simulink model "simulation_w_switch_sln3"  (Simulink 10.1)
settings: Solver=VariableStepAuto  StartTime=0.0  StopTime=tTot  MaxStep=1e-5  RelTol=1e-5
PreLoadFcn:
  | syst_init
values from neighbouring files (symbols this model uses):
  Aij = Aconn-Aii    [syst_init.m]
  AL = blkdiag(DGU.ALi)    [syst_init.m]
  atk24 = [zeros(3,1); 0.1*rand(3,1)-0.05]    [syst_init.m]
  atk34 = [zeros(3,1); 0.1*rand(3,1)-0.05]    [syst_init.m]
  B = blkdiag(DGU.B)    [syst_init.m]
  bC = blkdiag(DGU.bC)    [syst_init.m]
  bF = blkdiag(DGU.bF)    [syst_init.m]
  bH = blkdiag(DGU.bH)    [syst_init.m]
  bigCyComm = [zeros(3,3)  eye(3) zeros(3,30) ... (first row only)    [syst_init.m]
  bKhat = blkdiag(DGU.bKhat)    [syst_init.m]
  DGU = stateDyn(DGU,6)    [syst_init.m]
  F = blkdiag(DGU.Fj)    [syst_init.m]
  H = blkdiag(DGU.Hj)    [syst_init.m]
  K = blkdiag(DGU.K)    [syst_init.m]
  Khat = blkdiag(DGU.Khat)    [syst_init.m]
  L = blkdiag(DGU.Li)    [syst_init.m]
  n = 3    [syst_init.m]
  N = 6    [syst_init.m]
  nMaxMeas = .01    (= 0.01)    [syst_init.m]
  rhoMax = nMaxMeas*repmat([ones(n-1,1);0],N,1)    [syst_init.m]
  T = blkdiag(DGU.Tj)    [syst_init.m]
  Ta = 8    [syst_init.m]
  Tc = 2    [syst_init.m]
  tSampData = 1e-3    (= 0.001)    [syst_init.m]
  Vs = 60    [syst_init.m]
  wMax = nMax*repmat([ones(n-1,1);0],N,1)+nMaxMeas*repmat([zeros(n-1,1);1],N,1)    [syst_init.m]
undefined symbols (not defined in the file or in its folder): epsilon0bar, integral_Loc, rLoc_bar
libraries: powerlib x136, powerlib_meascontrol x13
(part 3 of 4)

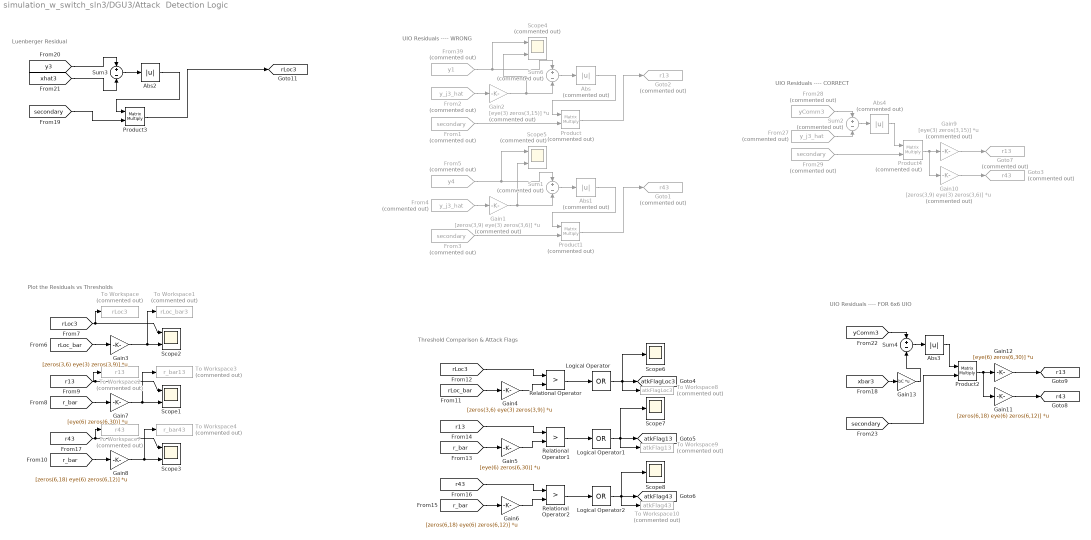
== system simulation_w_switch_sln3/DGU3/Attack  Detection Logic ==
  note: Luenberger Residual
  note: UIO Residuals ---- WRONG
  note: Threshold Comparison & Attack Flags
  note: Plot the Residuals vs Thresholds
  note: UIO Residuals ---- CORRECT
  note: UIO Residuals ---- FOR 6x6 UIO
  Abs : Abs  Commented=on
  Abs1 : Abs  Commented=on
  Abs2 : Abs
  Abs3 : Abs  ZeroCross=off
  Abs4 : Abs  Commented=on
  From1 : From  Commented=on  GotoTag=secondary  TagVisibility=global
  From2 : From  Commented=on  GotoTag=y_j3_hat  TagVisibility=global
  From27 : From  Commented=on  GotoTag=y_j3_hat  TagVisibility=global
  From28 : From  Commented=on  GotoTag=yComm3  TagVisibility=global
  From29 : From  Commented=on  GotoTag=secondary  TagVisibility=global
  From3 : From  Commented=on  GotoTag=secondary  TagVisibility=global
  From39 : From  Commented=on  GotoTag=y1  TagVisibility=global
  From4 : From  Commented=on  GotoTag=y_j3_hat  TagVisibility=global
  From5 : From  Commented=on  GotoTag=y4  TagVisibility=global
  Gain1 : Gain  Commented=on  Gain=[zeros(3,9) eye(3) zeros(3,6)]  Multiplication=Matrix(K*u) (u vector)
  Gain10 : Gain  Commented=on  Gain=[zeros(3,9) eye(3) zeros(3,6)]  Multiplication=Matrix(K*u) (u vector)
  Gain11 : Gain  Gain=[zeros(6,18) eye(6) zeros(6,12)]  Multiplication=Matrix(K*u) (u vector)
  Gain12 : Gain  Gain=[eye(6) zeros(6,30)]  Multiplication=Matrix(K*u) (u vector)
  Gain13 : Gain  Gain=bC  Multiplication=Matrix(K*u) (u vector)
  Gain2 : Gain  Commented=on  Gain=[eye(3) zeros(3,15)]  Multiplication=Matrix(K*u) (u vector)
  Gain3 : Gain  Gain=[zeros(3,6) eye(3) zeros(3,9)]  Multiplication=Matrix(K*u) (u vector)
  Gain4 : Gain  Gain=[zeros(3,6) eye(3) zeros(3,9)]  Multiplication=Matrix(K*u) (u vector)
  Gain5 : Gain  Gain=[eye(6) zeros(6,30)]  Multiplication=Matrix(K*u) (u vector)
  Gain6 : Gain  Gain=[zeros(6,18) eye(6) zeros(6,12)]  Multiplication=Matrix(K*u) (u vector)
  Gain7 : Gain  Gain=[eye(6) zeros(6,30)]  Multiplication=Matrix(K*u) (u vector)
  Gain8 : Gain  Gain=[zeros(6,18) eye(6) zeros(6,12)]  Multiplication=Matrix(K*u) (u vector)
  Gain9 : Gain  Commented=on  Gain=[eye(3) zeros(3,15)]  Multiplication=Matrix(K*u) (u vector)
  Goto1 : Goto  Commented=on  GotoTag=r43  TagVisibility=global
  Goto2 : Goto  Commented=on  GotoTag=r13  TagVisibility=global
  Goto3 : Goto  Commented=on  GotoTag=r43  TagVisibility=global
  Goto7 : Goto  Commented=on  GotoTag=r13  TagVisibility=global
  Logical Operator : Logic  Operator=OR  Inputs=1  AllPortsSameDT=off  OutDataTypeStr=boolean
  Logical Operator1 : Logic  Operator=OR  Inputs=1  AllPortsSameDT=off  OutDataTypeStr=boolean
  Logical Operator2 : Logic  Operator=OR  Inputs=1  AllPortsSameDT=off  OutDataTypeStr=boolean
  Product : Product  Commented=on  Multiplication=Matrix(*)
  Product1 : Product  Commented=on  Multiplication=Matrix(*)
  Product2 : Product  Multiplication=Matrix(*)
  Product3 : Product  Multiplication=Matrix(*)
  Product4 : Product  Commented=on  Multiplication=Matrix(*)
  Relational Operator : RelationalOperator  Operator=>  OutDataTypeStr=boolean  RndMeth=Simplest
  Relational Operator1 : RelationalOperator  Operator=>  OutDataTypeStr=boolean  RndMeth=Simplest
  Relational Operator2 : RelationalOperator  Operator=>  OutDataTypeStr=boolean  RndMeth=Simplest
  Scope1 : Scope  NumInputPorts=2
  Scope2 : Scope  NumInputPorts=2
  Scope3 : Scope  NumInputPorts=2
  Scope4 : Scope  Commented=on  NumInputPorts=2
  Scope5 : Scope  Commented=on  NumInputPorts=2
  Scope6 : Scope
  Scope7 : Scope
  Scope8 : Scope
  Sum1 : Sum  Commented=on  Inputs=+|-
  Sum2 : Sum  Commented=on  Inputs=+|-
  Sum3 : Sum  Inputs=+|-
  Sum4 : Sum  Inputs=+|-
  Sum6 : Sum  Commented=on  Inputs=+|-
  To Workspace : ToWorkspace  Commented=on  VariableName=rLoc3  SaveFormat=Timeseries  SampleTime=tSampData
  To Workspace1 : ToWorkspace  Commented=on  VariableName=rLoc_bar3  SaveFormat=Timeseries  SampleTime=tSampData
  To Workspace10 : ToWorkspace  Commented=on  VariableName=atkFlag43  SaveFormat=Timeseries  SampleTime=tSampData
  To Workspace2 : ToWorkspace  Commented=on  VariableName=r13  SaveFormat=Timeseries  SampleTime=tSampData
  To Workspace3 : ToWorkspace  Commented=on  VariableName=r_bar13  SaveFormat=Timeseries  SampleTime=tSampData
  To Workspace4 : ToWorkspace  Commented=on  VariableName=r_bar43  SaveFormat=Timeseries  SampleTime=tSampData
  To Workspace7 : ToWorkspace  Commented=on  VariableName=r43  SaveFormat=Timeseries  SampleTime=tSampData
  To Workspace8 : ToWorkspace  Commented=on  VariableName=atkFlagLoc3  SaveFormat=Timeseries  SampleTime=tSampData
  To Workspace9 : ToWorkspace  Commented=on  VariableName=atkFlag13  SaveFormat=Timeseries  SampleTime=tSampData
  tag scope: atkFlag13=global, atkFlag43=global, atkFlagLoc3=global, r13=global, r43=global, rLoc3=global
  wires:
  Abs2/1 -> Product3/1
  [secondary] -> Product3/2
  [xhat3] -> Sum3/2
  Sum3/1 -> Abs2/1
  Product3/1 -> [rLoc3]
  [y3] -> Sum3/1
  Gain2/1 -> Scope4/2, Sum6/2
  Sum1/1 -> Abs1/1
  Sum6/1 -> Abs/1
  Product1/1 -> Goto1/1
  Abs1/1 -> Product1/1
  From5/1 -> Scope5/1, Sum1/1
  From2/1 -> Gain2/1
  From4/1 -> Gain1/1
  From1/1 -> Product/2
  Gain1/1 -> Scope5/2, Sum1/2
  From3/1 -> Product1/2
  Abs/1 -> Product/1
  Product/1 -> Goto2/1
  From39/1 -> Scope4/1, Sum6/1
  Relational Operator1/1 -> Logical Operator1/1
  [rLoc_bar] -> Gain4/1
  Logical Operator1/1 -> Scope7/1, To Workspace9/1, [atkFlag13]
  [rLoc3] -> Relational Operator/1
  Relational Operator/1 -> Logical Operator/1
  [r_bar] -> Gain5/1
  Gain5/1 -> Relational Operator1/2
  Logical Operator/1 -> Scope6/1, To Workspace8/1, [atkFlagLoc3]
  [r13] -> Relational Operator1/1
  Relational Operator2/1 -> Logical Operator2/1
  Gain4/1 -> Relational Operator/2
  Gain6/1 -> Relational Operator2/2
  [r43] -> Relational Operator2/1
  [r_bar] -> Gain6/1
  Logical Operator2/1 -> Scope8/1, To Workspace10/1, [atkFlag43]
  [r_bar] -> Gain8/1
  [r43] -> To Workspace7/1, Scope3/1
  [r13] -> To Workspace2/1, Scope1/1
  [r_bar] -> Gain7/1
  Gain7/1 -> To Workspace3/1, Scope1/2
  [rLoc_bar] -> Gain3/1
  Gain3/1 -> To Workspace1/1, Scope2/2
  Gain8/1 -> To Workspace4/1, Scope3/2
  [rLoc3] -> To Workspace/1, Scope2/1
  From29/1 -> Product4/2
  From27/1 -> Sum2/2
  From28/1 -> Sum2/1
  Sum2/1 -> Abs4/1
  Product4/1 -> Gain10/1, Gain9/1
  Abs4/1 -> Product4/1
  Gain9/1 -> Goto7/1
  Gain10/1 -> Goto3/1
  Gain11/1 -> [r43]
  Gain12/1 -> [r13]
  Abs3/1 -> Product2/1
  Product2/1 -> Gain12/1, Gain11/1
  Sum4/1 -> Abs3/1
  [yComm3] -> Sum4/1
  [secondary] -> Product2/2
  [xbar3] -> Gain13/1
  Gain13/1 -> Sum4/2

== system simulation_w_switch_sln3/DGU3/Luenberger  Observer ==
  Gain1 : Gain  Gain=bigCyComm  Multiplication=Matrix(K*u) (u vector)
  Gain17 : Gain  Gain=[DGU(3).B , DGU(3).Li , DGU(3).M , Aij(2*n+1:3*n,:)]  Multiplication=Matrix(K*u) (u vector)
  Gain18 : Gain  Gain=DGU(3).A-DGU(3).Li*DGU(3).C  Multiplication=Matrix(K*u) (u vector)
  Integrator4 : Integrator  ExternalReset=rising  InitialConditionSource=external  InitialCondition=[0;0;0]
  Mux : Mux  Inputs=5
  Product4 : Product  Multiplication=Matrix(*)
  Sum10 : Sum  Inputs=++|
  tag scope: xhat3=global
  wires:
  Product4/1 -> [xhat3]
  [Il3] -> Mux/3
  [y3] -> Integrator4/3, Mux/2
  [Vref3] -> Mux/4
  Gain17/1 -> Sum10/2
  Gain18/1 -> Sum10/1
  [secondary] -> Integrator4/2, Product4/2
  Mux/1 -> Gain17/1
  Sum10/1 -> Integrator4/1
  Integrator4/1 -> Product4/1, Gain18/1
  [Vt3] -> Mux/1
  [yComm3] -> Gain1/1
  Gain1/1 -> Mux/5

== system simulation_w_switch_sln3/DGU3/Primary  Voltage  Controller ==
  Gain1 : Gain  Gain=DGU(3).K  Multiplication=Matrix(K*u) (u vector)
  tag scope: Vt3d=global
  wires:
  Gain1/1 -> [Vt3d]
  [y3] -> Gain1/1

== system simulation_w_switch_sln3/DGU3/Secondary  Consensus Layer ==
  note: deltaV3
  Gain14 : Gain  Gain=DGU(3).kI
  Gain2 : Gain  Gain=repmat([0 0 0 0 1 0],1,6)  Multiplication=Matrix(K*u) (u vector)
  Gain8 : Gain  Gain=length(DGU(3).Ni)
  Integrator2 : Integrator  ExternalReset=rising
  Sum10 : Sum  Inputs=|+-
  Sum11 : Sum  Inputs=|++
  Switch2 : Switch  Criteria=u2 > Threshold  Threshold=0.1
  tag scope: Vref3=global
  wires:
  Gain8/1 -> Sum10/2
  [It3] -> Gain8/1
  Integrator2/1 -> Sum11/1
  [secondary] -> Integrator2/2, Switch2/2
  Gain2/1 -> Sum10/1
  [yComm3] -> Gain2/1
  Sum10/1 -> Gain14/1
  Gain14/1 -> Integrator2/1
  Switch2/1 -> [Vref3]
  Sum11/1 -> Switch2/1
  [Vref] -> Switch2/3, Sum11/2

== system simulation_w_switch_sln3/DGU3/Switching ==
  Divide : Product  Inputs=*/
  Logical Operator : Logic  Operator=NOT  AllPortsSameDT=off  OutDataTypeStr=boolean
  PWM Generator (DC-DC) : powerlib_meascontrol/Pulse & Signal Generators/PWM Generator (DC-DC)  Fsw=10000  Ts=0
  tag scope: SW_Buck_3=global, SW_Buck_3n=global, SW_Duty_3=global
  wires:
  [Vs3] -> Divide/2
  Logical Operator/1 -> [SW_Buck_3n]
  PWM Generator (DC-DC)/1 -> Logical Operator/1, [SW_Buck_3]
  Divide/1 -> [SW_Duty_3], PWM Generator (DC-DC)/1
  [Vt3d] -> Divide/1

== system simulation_w_switch_sln3/DGU3/UIO ==
  note: Single UIO for all neighbors of DGU 1 with Switched Inputs
  note: Calculated Switching Inputs
  note: 6x6 UIO for the states of DGUs with average dynamics
  Constant1 : Constant  Commented=on  Value=Vs
  Constant2 : Constant  Commented=on  Value=0.8132
  Divide : Product  Commented=on  Inputs=*/  Multiplication=Matrix(*)
  From5 : From  Commented=on  GotoTag=yComm3  TagVisibility=global
  From7 : From  Commented=on  GotoTag=yComm3  TagVisibility=global
  From8 : From  Commented=on  GotoTag=SW_yComm3  TagVisibility=global
  From9 : From  Commented=on  GotoTag=secondary  TagVisibility=global
  Gain15 : Gain  Gain=bH  Multiplication=Matrix(K*u) (u vector)
  Gain16 : Gain  Gain=inv(bC)-bH  Multiplication=Matrix(K*u) (u vector)
  Gain17 : Gain  Gain=bKhat  Multiplication=Matrix(K*u) (u vector)
  Gain18 : Gain  Gain=bF  Multiplication=Matrix(K*u) (u vector)
  Gain4 : Gain  Commented=on  Gain=K  Multiplication=Matrix(K*u) (u vector)
  Gain5 : Gain  Commented=on  Gain=[Khat T*B]  Multiplication=Matrix(K*u) (u vector)
  Gain6 : Gain  Commented=on  Gain=F  Multiplication=Matrix(K*u) (u vector)
  Gain7 : Gain  Commented=on  Gain=59.7999
  Gain8 : Gain  Commented=on  Gain=H  Multiplication=Matrix(K*u) (u vector)
  Gain9 : Gain  Commented=on  Gain=T  Multiplication=Matrix(K*u) (u vector)
  Goto : Goto  Commented=on  GotoTag=SW_yComm3  TagVisibility=global
  Goto3 : Goto  Commented=on  GotoTag=y_j3_hat  TagVisibility=global
  Goto4 : Goto  Commented=on  GotoTag=Duty_yComm3  TagVisibility=global
  Integrator1 : Integrator  Commented=on  ExternalReset=rising  InitialConditionSource=external
  Integrator4 : Integrator  ExternalReset=rising  InitialConditionSource=external  InitialCondition=[0;0;0]
  Mux3 : Mux  Commented=on  Inputs=2
  PWM Generator (DC-DC) : powerlib_meascontrol/Pulse & Signal Generators/PWM Generator (DC-DC)  Commented=on  Fsw=10000  Ts=0
  Product1 : Product  Commented=on  Multiplication=Matrix(*)
  Product4 : Product  Multiplication=Matrix(*)
  Sum10 : Sum  Inputs=++|
  Sum11 : Sum  Inputs=++|
  Sum2 : Sum  Commented=on  Inputs=++|
  Sum3 : Sum  Commented=on  Inputs=++|
  Sum4 : Sum  Commented=on  Inputs=|-+
  tag scope: xbar3=global
  wires:
  PWM Generator (DC-DC)/1 -> Goto/1
  Divide/1 -> Goto4/1, PWM Generator (DC-DC)/1
  Constant1/1 -> Divide/2
  Gain4/1 -> Divide/1
  From7/1 -> Gain4/1
  Constant2/1 -> Sum4/1
  From5/1 -> Gain8/1, Gain9/1, Mux3/1
  Sum3/1 -> Product1/1
  Gain5/1 -> Sum2/2
  Gain7/1 -> Sum4/2
  From8/1 -> Gain7/1
  Mux3/1 -> Gain5/1
  Gain8/1 -> Sum3/1
  Gain9/1 -> Integrator1/3
  From9/1 -> Integrator1/2, Product1/2
  Sum2/1 -> Integrator1/1
  Sum4/1 -> Mux3/2
  Integrator1/1 -> Sum3/2, Gain6/1
  Gain6/1 -> Sum2/1
  Product1/1 -> Goto3/1
  Gain17/1 -> Sum10/2
  Gain18/1 -> Sum10/1
  [secondary] -> Integrator4/2, Product4/2
  Product4/1 -> [xbar3]
  Integrator4/1 -> Sum11/2, Gain18/1
  Gain15/1 -> Sum11/1
  Sum10/1 -> Integrator4/1
  [yComm3] -> Gain16/1, Gain15/1, Gain17/1
  Gain16/1 -> Integrator4/3
  Sum11/1 -> Product4/1

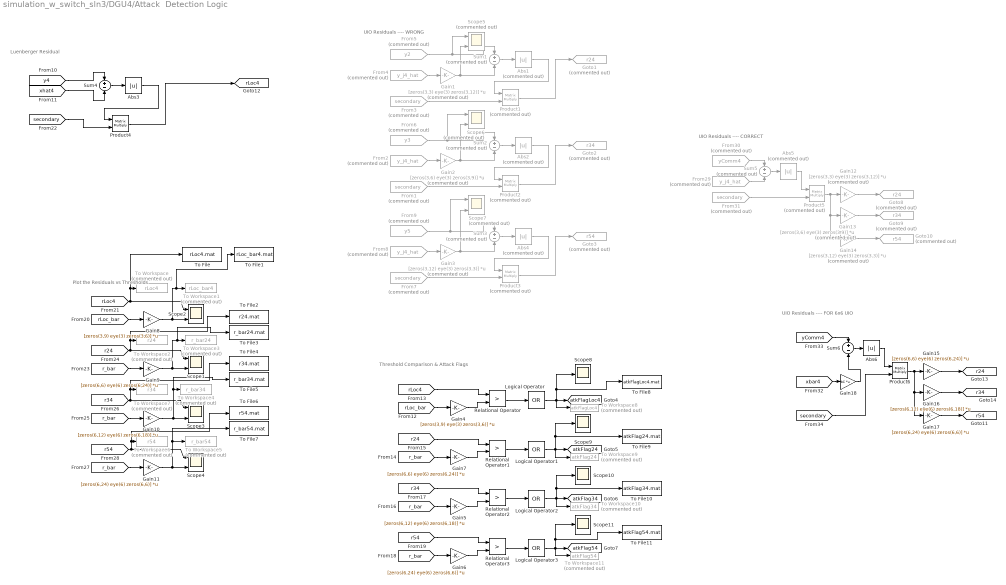
== system simulation_w_switch_sln3/DGU4/Attack  Detection Logic ==
  note: UIO Residuals ---- WRONG
  note: Luenberger Residual
  note: Threshold Comparison & Attack Flags
  note: Plot the Residuals vs Thresholds
  note: UIO Residuals ---- CORRECT
  note: UIO Residuals ---- FOR 6x6 UIO
  Abs{1..2,4..5} (4 alike) : Abs  Commented=on
  Abs3 : Abs
  Abs6 : Abs  ZeroCross=off
  From{1,3,7,31} (4 alike) : From  Commented=on  GotoTag=secondary  TagVisibility=global
  From{2,4,8,29} (4 alike) : From  Commented=on  GotoTag=y_j4_hat  TagVisibility=global
  From30 : From  Commented=on  GotoTag=yComm4  TagVisibility=global
  From5 : From  Commented=on  GotoTag=y2  TagVisibility=global
  From6 : From  Commented=on  GotoTag=y3  TagVisibility=global
  From9 : From  Commented=on  GotoTag=y5  TagVisibility=global
  Gain1 : Gain  Commented=on  Gain=[zeros(3,3) eye(3) zeros(3,12)]  Multiplication=Matrix(K*u) (u vector)
  Gain10 : Gain  Gain=[zeros(6,12) eye(6) zeros(6,18)]  Multiplication=Matrix(K*u) (u vector)
  Gain11 : Gain  Gain=[zeros(6,24) eye(6) zeros(6,6)]  Multiplication=Matrix(K*u) (u vector)
  Gain12 : Gain  Commented=on  Gain=[zeros(3,3) eye(3) zeros(3,12)]  Multiplication=Matrix(K*u) (u vector)
  Gain13 : Gain  Commented=on  Gain=[zeros(3,6) eye(3) zeros(3,9)]  Multiplication=Matrix(K*u) (u vector)
  Gain14 : Gain  Commented=on  Gain=[zeros(3,12) eye(3) zeros(3,3)]  Multiplication=Matrix(K*u) (u vector)
  Gain15 : Gain  Gain=[zeros(6,6) eye(6) zeros(6,24)]  Multiplication=Matrix(K*u) (u vector)
  Gain16 : Gain  Gain=[zeros(6,12) eye(6) zeros(6,18)]  Multiplication=Matrix(K*u) (u vector)
  Gain17 : Gain  Gain=[zeros(6,24) eye(6) zeros(6,6)]  Multiplication=Matrix(K*u) (u vector)
  Gain18 : Gain  Gain=bC  Multiplication=Matrix(K*u) (u vector)
  Gain2 : Gain  Commented=on  Gain=[zeros(3,6) eye(3) zeros(3,9)]  Multiplication=Matrix(K*u) (u vector)
  Gain3 : Gain  Commented=on  Gain=[zeros(3,12) eye(3) zeros(3,3)]  Multiplication=Matrix(K*u) (u vector)
  Gain4 : Gain  Gain=[zeros(3,9) eye(3) zeros(3,6)]  Multiplication=Matrix(K*u) (u vector)
  Gain5 : Gain  Gain=[zeros(6,12) eye(6) zeros(6,18)]  Multiplication=Matrix(K*u) (u vector)
  Gain6 : Gain  Gain=[zeros(6,24) eye(6) zeros(6,6)]  Multiplication=Matrix(K*u) (u vector)
  Gain7 : Gain  Gain=[zeros(6,6) eye(6) zeros(6,24)]  Multiplication=Matrix(K*u) (u vector)
  Gain8 : Gain  Gain=[zeros(3,9) eye(3) zeros(3,6)]  Multiplication=Matrix(K*u) (u vector)
  Gain9 : Gain  Gain=[zeros(6,6) eye(6) zeros(6,24)]  Multiplication=Matrix(K*u) (u vector)
  Goto1 : Goto  Commented=on  GotoTag=r24  TagVisibility=global
  Goto10 : Goto  Commented=on  GotoTag=r54  TagVisibility=global
  Goto2 : Goto  Commented=on  GotoTag=r34  TagVisibility=global
  Goto3 : Goto  Commented=on  GotoTag=r54  TagVisibility=global
  Goto8 : Goto  Commented=on  GotoTag=r24  TagVisibility=global
  Goto9 : Goto  Commented=on  GotoTag=r34  TagVisibility=global
  Logical Operator{,1..3} (4 alike) : Logic  Operator=OR  Inputs=1  AllPortsSameDT=off  OutDataTypeStr=boolean
  Product{1..3,5} (4 alike) : Product  Commented=on  Multiplication=Matrix(*)
  Product4 : Product  Multiplication=Matrix(*)
  Product6 : Product  Multiplication=Matrix(*)
  Relational Operator{,1..3} (4 alike) : RelationalOperator  Operator=>  OutDataTypeStr=boolean  RndMeth=Simplest
  Scope{1..4} (4 alike) : Scope  NumInputPorts=2
  Scope{8..11} (4 alike) : Scope
  Scope5 : Scope  Commented=on  NumInputPorts=2
  Scope6 : Scope  Commented=on  NumInputPorts=2
  Scope7 : Scope  Commented=on  NumInputPorts=2
  Sum{1..3,5} (4 alike) : Sum  Commented=on  Inputs=+|-
  Sum4 : Sum  Inputs=+|-
  Sum6 : Sum  Inputs=+|-
  To File : ToFile  Filename=rLoc4.mat  MatrixName=rLoc4  SaveFormat=Timeseries  SampleTime=tSampData
  To File1 : ToFile  Filename=rLoc_bar4.mat  MatrixName=rLoc_bar4  SaveFormat=Timeseries  SampleTime=tSampData
  To File10 : ToFile  Filename=atkFlag34.mat  MatrixName=atkFlag34  SaveFormat=Timeseries  SampleTime=tSampData
  To File11 : ToFile  Filename=atkFlag54.mat  MatrixName=atkFlag54  SaveFormat=Timeseries  SampleTime=tSampData
  To File2 : ToFile  Filename=r24.mat  MatrixName=r24  SaveFormat=Timeseries  SampleTime=tSampData
  To File3 : ToFile  Filename=r_bar24.mat  MatrixName=r_bar24  SaveFormat=Timeseries  SampleTime=tSampData
  To File4 : ToFile  Filename=r34.mat  MatrixName=r34  SaveFormat=Timeseries  SampleTime=tSampData
  To File5 : ToFile  Filename=r_bar34.mat  MatrixName=r_bar34  SaveFormat=Timeseries  SampleTime=tSampData
  To File6 : ToFile  Filename=r54.mat  MatrixName=r54  SaveFormat=Timeseries  SampleTime=tSampData
  To File7 : ToFile  Filename=r_bar54.mat  MatrixName=r_bar54  SaveFormat=Timeseries  SampleTime=tSampData
  To File8 : ToFile  Filename=atkFlagLoc4.mat  MatrixName=atkFlagLoc4  SaveFormat=Timeseries  SampleTime=tSampData
  To File9 : ToFile  Filename=atkFlag24.mat  MatrixName=atkFlag24  SaveFormat=Timeseries  SampleTime=tSampData
  To Workspace : ToWorkspace  Commented=on  VariableName=rLoc4  SaveFormat=Timeseries  SampleTime=tSampData
  To Workspace1 : ToWorkspace  Commented=on  VariableName=rLoc_bar4  SaveFormat=Timeseries  SampleTime=tSampData
  To Workspace10 : ToWorkspace  Commented=on  VariableName=atkFlag34  SaveFormat=Timeseries  SampleTime=tSampData
  To Workspace11 : ToWorkspace  Commented=on  VariableName=atkFlag54  SaveFormat=Timeseries  SampleTime=tSampData
  To Workspace2 : ToWorkspace  Commented=on  VariableName=r24  SaveFormat=Timeseries  SampleTime=tSampData
  To Workspace3 : ToWorkspace  Commented=on  VariableName=r_bar24  SaveFormat=Timeseries  SampleTime=tSampData
  To Workspace4 : ToWorkspace  Commented=on  VariableName=r_bar34  SaveFormat=Timeseries  SampleTime=tSampData
  To Workspace5 : ToWorkspace  Commented=on  VariableName=r_bar54  SaveFormat=Timeseries  SampleTime=tSampData
  To Workspace6 : ToWorkspace  Commented=on  VariableName=r54  SaveFormat=Timeseries  SampleTime=tSampData
  To Workspace7 : ToWorkspace  Commented=on  VariableName=r34  SaveFormat=Timeseries  SampleTime=tSampData
  To Workspace8 : ToWorkspace  Commented=on  VariableName=atkFlagLoc4  SaveFormat=Timeseries  SampleTime=tSampData
  To Workspace9 : ToWorkspace  Commented=on  VariableName=atkFlag24  SaveFormat=Timeseries  SampleTime=tSampData
  tag scope: atkFlag24=global, atkFlag34=global, atkFlag54=global, atkFlagLoc4=global, r24=global, r34=global, r54=global, rLoc4=global
  wires:
  [secondary] -> Product4/2
  Product4/1 -> [rLoc4]
  Abs3/1 -> Product4/1
  [y4] -> Sum4/1
  Sum4/1 -> Abs3/1
  [xhat4] -> Sum4/2
  Gain1/1 -> Scope5/2, Sum1/2
  Abs1/1 -> Product1/1
  Product1/1 -> Goto1/1
  From3/1 -> Product1/2
  Sum1/1 -> Abs1/1
  From4/1 -> Gain1/1
  From6/1 -> Scope6/1, Sum2/1
  Abs2/1 -> Product2/1
  From1/1 -> Product2/2
  Product2/1 -> Goto2/1
  Gain2/1 -> Scope6/2, Sum2/2
  From2/1 -> Gain2/1
  Sum2/1 -> Abs2/1
  From9/1 -> Scope7/1, Sum3/1
  Abs4/1 -> Product3/1
  From7/1 -> Product3/2
  Product3/1 -> Goto3/1
  Gain3/1 -> Scope7/2, Sum3/2
  From8/1 -> Gain3/1
  Sum3/1 -> Abs4/1
  Logical Operator3/1 -> To Workspace11/1, Scope11/1, To File11/1, [atkFlag54]
  Relational Operator1/1 -> Logical Operator1/1
  [rLoc_bar] -> Gain4/1
  [r_bar] -> Gain6/1
  Logical Operator1/1 -> To Workspace9/1, To File9/1, Scope9/1, [atkFlag24]
  [r54] -> Relational Operator3/1
  [rLoc4] -> Relational Operator/1
  Relational Operator/1 -> Logical Operator/1
  Gain6/1 -> Relational Operator3/2
  [r_bar] -> Gain7/1
  Gain7/1 -> Relational Operator1/2
  Logical Operator/1 -> To Workspace8/1, To File8/1, Scope8/1, [atkFlagLoc4]
  Relational Operator3/1 -> Logical Operator3/1
  [r24] -> Relational Operator1/1
  Relational Operator2/1 -> Logical Operator2/1
  Gain4/1 -> Relational Operator/2
  Gain5/1 -> Relational Operator2/2
  [r34] -> Relational Operator2/1
  [r_bar] -> Gain5/1
  Logical Operator2/1 -> To Workspace10/1, Scope10/1, To File10/1, [atkFlag34]
  [rLoc_bar] -> Gain8/1
  [r_bar] -> Gain9/1
  [r54] -> To File6/1, To Workspace6/1, Scope4/1
  [r_bar] -> Gain10/1
  Gain11/1 -> To File7/1, To Workspace5/1, Scope4/2
  [rLoc4] -> To File/1, To Workspace/1, Scope2/1
  [r_bar] -> Gain11/1
  Gain9/1 -> To File3/1, To Workspace3/1, Scope1/2
  [r34] -> To File4/1, To Workspace7/1, Scope3/1
  Gain10/1 -> To File5/1, To Workspace4/1, Scope3/2
  Gain8/1 -> To File1/1, To Workspace1/1, Scope2/2
  [r24] -> To File2/1, To Workspace2/1, Scope1/1
  From5/1 -> Scope5/1, Sum1/1
  From31/1 -> Product5/2
  From29/1 -> Sum5/2
  From30/1 -> Sum5/1
  Sum5/1 -> Abs5/1
  Product5/1 -> Gain12/1, Gain14/1, Gain13/1
  Abs5/1 -> Product5/1
  Gain14/1 -> Goto10/1
  Gain13/1 -> Goto9/1
  Gain12/1 -> Goto8/1
  Gain15/1 -> [r24]
  Gain16/1 -> [r34]
  Gain17/1 -> [r54]
  Abs6/1 -> Product6/1
  Product6/1 -> Gain16/1, Gain17/1, Gain15/1
  Sum6/1 -> Abs6/1
  [yComm4] -> Sum6/1
  [secondary] -> Product6/2
  [xbar4] -> Gain18/1
  Gain18/1 -> Sum6/2

== system simulation_w_switch_sln3/DGU4/Luenberger  Observer ==
  Gain1 : Gain  Gain=bigCyComm  Multiplication=Matrix(K*u) (u vector)
  Gain17 : Gain  Gain=[DGU(4).B , DGU(4).Li , DGU(4).M , Aij(3*n+1:4*n,:)]  Multiplication=Matrix(K*u) (u vector)
  Gain18 : Gain  Gain=DGU(4).A-DGU(4).Li*DGU(4).C  Multiplication=Matrix(K*u) (u vector)
  Integrator4 : Integrator  ExternalReset=rising  InitialConditionSource=external  InitialCondition=[0;0;0]
  Mux : Mux  Inputs=5
  Product4 : Product  Multiplication=Matrix(*)
  Sum10 : Sum  Inputs=++|
  tag scope: xhat4=global
  wires:
  Product4/1 -> [xhat4]
  [Il4] -> Mux/3
  [y4] -> Integrator4/3, Mux/2
  [Vref4] -> Mux/4
  Gain17/1 -> Sum10/2
  Gain18/1 -> Sum10/1
  [secondary] -> Integrator4/2, Product4/2
  Mux/1 -> Gain17/1
  Sum10/1 -> Integrator4/1
  Integrator4/1 -> Product4/1, Gain18/1
  [Vt4] -> Mux/1
  [yComm4] -> Gain1/1
  Gain1/1 -> Mux/5

== system simulation_w_switch_sln3/DGU4/Primary  Voltage  Controller ==
  Gain1 : Gain  Gain=DGU(4).K  Multiplication=Matrix(K*u) (u vector)
  tag scope: Vt4d=global
  wires:
  Gain1/1 -> [Vt4d]
  [y4] -> Gain1/1

== system simulation_w_switch_sln3/DGU4/Secondary Consensus Layer ==
  note: deltaV4
  Gain15 : Gain  Gain=DGU(4).kI
  Gain3 : Gain  Gain=repmat([0 0 0 0 1 0],1,6)  Multiplication=Matrix(K*u) (u vector)
  Gain9 : Gain  Gain=length(DGU(4).Ni)
  Integrator3 : Integrator  ExternalReset=rising
  Sum12 : Sum  Inputs=|+-
  Sum13 : Sum  Inputs=|++
  Switch3 : Switch  Criteria=u2 > Threshold  Threshold=0.1
  tag scope: Vref4=global
  wires:
  Gain3/1 -> Sum12/1
  Switch3/1 -> [Vref4]
  Integrator3/1 -> Sum13/1
  [It4] -> Gain9/1
  Sum12/1 -> Gain15/1
  Sum13/1 -> Switch3/1
  Gain15/1 -> Integrator3/1
  [secondary] -> Integrator3/2, Switch3/2
  [Vref] -> Switch3/3, Sum13/2
  [yComm4] -> Gain3/1
  Gain9/1 -> Sum12/2

== system simulation_w_switch_sln3/DGU4/Switching ==
  Divide : Product  Inputs=*/
  Logical Operator : Logic  Operator=NOT  AllPortsSameDT=off  OutDataTypeStr=boolean
  PWM Generator (DC-DC) : powerlib_meascontrol/Pulse & Signal Generators/PWM Generator (DC-DC)  Fsw=10000  Ts=0
  tag scope: SW_Buck_4=global, SW_Buck_4n=global, SW_Duty_4=global
  wires:
  [Vs4] -> Divide/2
  Logical Operator/1 -> [SW_Buck_4n]
  PWM Generator (DC-DC)/1 -> Logical Operator/1, [SW_Buck_4]
  Divide/1 -> [SW_Duty_4], PWM Generator (DC-DC)/1
  [Vt4d] -> Divide/1

== system simulation_w_switch_sln3/DGU4/UIO ==
  note: Single UIO for all neighbors of DGU 1 with Switched Inputs
  note: Calculated Switching Inputs
  note: 6x6 UIO for the states of DGUs with average dynamics
  Constant1 : Constant  Commented=on  Value=Vs
  Constant2 : Constant  Commented=on  Value=0.8132
  Divide : Product  Commented=on  Inputs=*/  Multiplication=Matrix(*)
  From1 : From  Commented=on  GotoTag=u_SW_a2  TagVisibility=global
  From5 : From  Commented=on  GotoTag=yComm4  TagVisibility=global
  From7 : From  Commented=on  GotoTag=yComm4  TagVisibility=global
  From8 : From  Commented=on  GotoTag=SW_yComm4  TagVisibility=global
  From9 : From  Commented=on  GotoTag=secondary  TagVisibility=global
  Gain1 : Gain  Commented=on  Gain=[0 1 0 0 0 0]  Multiplication=Matrix(K*u) (u vector)
  Gain15 : Gain  Gain=bH  Multiplication=Matrix(K*u) (u vector)
  Gain16 : Gain  Gain=inv(bC)-bH  Multiplication=Matrix(K*u) (u vector)
  Gain17 : Gain  Gain=bKhat  Multiplication=Matrix(K*u) (u vector)
  Gain18 : Gain  Gain=bF  Multiplication=Matrix(K*u) (u vector)
  Gain4 : Gain  Commented=on  Gain=K  Multiplication=Matrix(K*u) (u vector)
  Gain5 : Gain  Commented=on  Gain=[Khat T*B]  Multiplication=Matrix(K*u) (u vector)
  Gain6 : Gain  Commented=on  Gain=F  Multiplication=Matrix(K*u) (u vector)
  Gain7 : Gain  Commented=on  Gain=59.7999
  Gain8 : Gain  Commented=on  Gain=H  Multiplication=Matrix(K*u) (u vector)
  Gain9 : Gain  Commented=on  Gain=T  Multiplication=Matrix(K*u) (u vector)
  Goto : Goto  Commented=on  GotoTag=SW_yComm4  TagVisibility=global
  Goto3 : Goto  Commented=on  GotoTag=y_j4_hat  TagVisibility=global
  Goto4 : Goto  Commented=on  GotoTag=Duty_yComm4  TagVisibility=global
  Integrator1 : Integrator  Commented=on  ExternalReset=rising  InitialConditionSource=external
  Integrator4 : Integrator  ExternalReset=rising  InitialConditionSource=external  InitialCondition=[0;0;0]
  Mux3 : Mux  Commented=on  Inputs=2
  PWM Generator (DC-DC) : powerlib_meascontrol/Pulse & Signal Generators/PWM Generator (DC-DC)  Commented=on  Fsw=10000  Ts=0
  Product1 : Product  Commented=on  Multiplication=Matrix(*)
  Product4 : Product  Multiplication=Matrix(*)
  Scope : Scope  Commented=on
  Sum1 : Sum  Commented=on  Inputs=+-|
  Sum10 : Sum  Inputs=++|
  Sum11 : Sum  Inputs=++|
  Sum2 : Sum  Commented=on  Inputs=++|
  Sum3 : Sum  Commented=on  Inputs=++|
  Sum4 : Sum  Commented=on  Inputs=|-+
  tag scope: xbar4=global
  wires:
  PWM Generator (DC-DC)/1 -> Goto/1
  Divide/1 -> Goto4/1, PWM Generator (DC-DC)/1
  Constant1/1 -> Divide/2
  Gain4/1 -> Divide/1
  From7/1 -> Gain4/1
  Constant2/1 -> Sum4/1
  From5/1 -> Gain8/1, Gain9/1, Mux3/1
  Sum3/1 -> Product1/1
  Gain5/1 -> Sum2/2
  Gain7/1 -> Sum4/2
  From8/1 -> Gain7/1
  Mux3/1 -> Gain5/1
  Gain8/1 -> Sum3/1
  Gain9/1 -> Integrator1/3
  From9/1 -> Integrator1/2, Product1/2
  Sum2/1 -> Integrator1/1
  Sum4/1 -> Gain1/1, Mux3/2
  Integrator1/1 -> Sum3/2, Gain6/1
  Gain6/1 -> Sum2/1
  Product1/1 -> Goto3/1
  Gain1/1 -> Sum1/1
  From1/1 -> Sum1/2
  Sum1/1 -> Scope/1
  Sum11/1 -> Product4/1
  Gain17/1 -> Sum10/2
  Gain16/1 -> Integrator4/3
  Sum10/1 -> Integrator4/1
  [yComm4] -> Gain16/1, Gain15/1, Gain17/1
  Gain18/1 -> Sum10/1
  Gain15/1 -> Sum11/1
  Product4/1 -> [xbar4]
  Integrator4/1 -> Sum11/2, Gain18/1
  [secondary] -> Integrator4/2, Product4/2

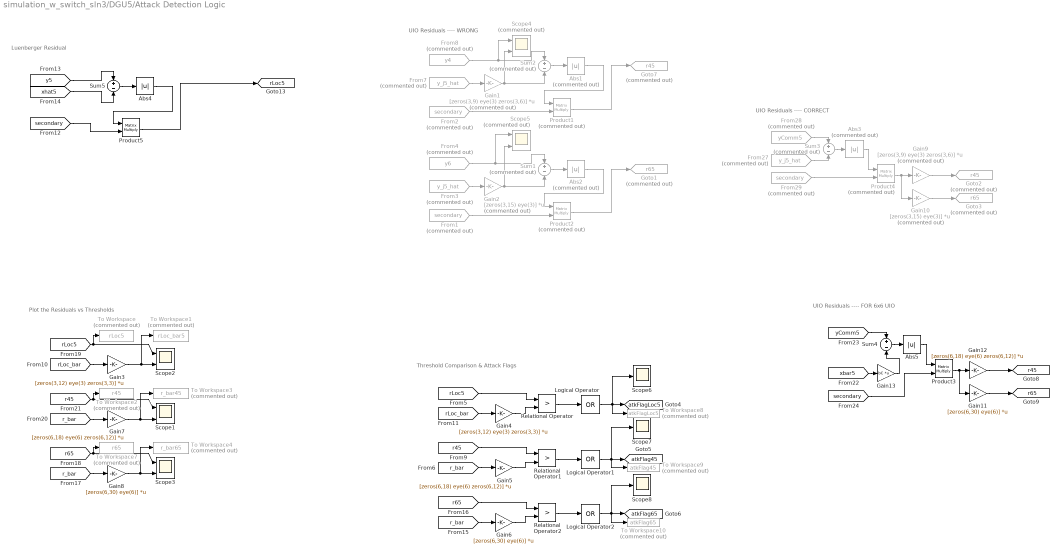
== system simulation_w_switch_sln3/DGU5/Attack Detection Logic ==
  note: UIO Residuals ---- WRONG
  note: Luenberger Residual
  note: Threshold Comparison & Attack Flags
  note: Plot the Residuals vs Thresholds
  note: UIO Residuals ---- CORRECT
  note: UIO Residuals ---- FOR 6x6 UIO
  Abs1 : Abs  Commented=on
  Abs2 : Abs  Commented=on
  Abs3 : Abs  Commented=on
  Abs4 : Abs
  Abs5 : Abs  ZeroCross=off
  From1 : From  Commented=on  GotoTag=secondary  TagVisibility=global
  From2 : From  Commented=on  GotoTag=secondary  TagVisibility=global
  From27 : From  Commented=on  GotoTag=y_j5_hat  TagVisibility=global
  From28 : From  Commented=on  GotoTag=yComm5  TagVisibility=global
  From29 : From  Commented=on  GotoTag=secondary  TagVisibility=global
  From3 : From  Commented=on  GotoTag=y_j5_hat  TagVisibility=global
  From4 : From  Commented=on  GotoTag=y6  TagVisibility=global
  From7 : From  Commented=on  GotoTag=y_j5_hat  TagVisibility=global
  From8 : From  Commented=on  GotoTag=y4  TagVisibility=global
  Gain1 : Gain  Commented=on  Gain=[zeros(3,9) eye(3) zeros(3,6)]  Multiplication=Matrix(K*u) (u vector)
  Gain10 : Gain  Commented=on  Gain=[zeros(3,15) eye(3)]  Multiplication=Matrix(K*u) (u vector)
  Gain11 : Gain  Gain=[zeros(6,30) eye(6)]  Multiplication=Matrix(K*u) (u vector)
  Gain12 : Gain  Gain=[zeros(6,18) eye(6) zeros(6,12)]  Multiplication=Matrix(K*u) (u vector)
  Gain13 : Gain  Gain=bC  Multiplication=Matrix(K*u) (u vector)
  Gain2 : Gain  Commented=on  Gain=[zeros(3,15) eye(3)]  Multiplication=Matrix(K*u) (u vector)
  Gain3 : Gain  Gain=[zeros(3,12) eye(3) zeros(3,3)]  Multiplication=Matrix(K*u) (u vector)
  Gain4 : Gain  Gain=[zeros(3,12) eye(3) zeros(3,3)]  Multiplication=Matrix(K*u) (u vector)
  Gain5 : Gain  Gain=[zeros(6,18) eye(6) zeros(6,12)]  Multiplication=Matrix(K*u) (u vector)
  Gain6 : Gain  Gain=[zeros(6,30) eye(6)]  Multiplication=Matrix(K*u) (u vector)
  Gain7 : Gain  Gain=[zeros(6,18) eye(6) zeros(6,12)]  Multiplication=Matrix(K*u) (u vector)
  Gain8 : Gain  Gain=[zeros(6,30) eye(6)]  Multiplication=Matrix(K*u) (u vector)
  Gain9 : Gain  Commented=on  Gain=[zeros(3,9) eye(3) zeros(3,6)]  Multiplication=Matrix(K*u) (u vector)
  Goto1 : Goto  Commented=on  GotoTag=r65  TagVisibility=global
  Goto2 : Goto  Commented=on  GotoTag=r45  TagVisibility=global
  Goto3 : Goto  Commented=on  GotoTag=r65  TagVisibility=global
  Goto7 : Goto  Commented=on  GotoTag=r45  TagVisibility=global
  Logical Operator : Logic  Operator=OR  Inputs=1  AllPortsSameDT=off  OutDataTypeStr=boolean
  Logical Operator1 : Logic  Operator=OR  Inputs=1  AllPortsSameDT=off  OutDataTypeStr=boolean
  Logical Operator2 : Logic  Operator=OR  Inputs=1  AllPortsSameDT=off  OutDataTypeStr=boolean
  Product1 : Product  Commented=on  Multiplication=Matrix(*)
  Product2 : Product  Commented=on  Multiplication=Matrix(*)
  Product3 : Product  Multiplication=Matrix(*)
  Product4 : Product  Commented=on  Multiplication=Matrix(*)
  Product5 : Product  Multiplication=Matrix(*)
  Relational Operator : RelationalOperator  Operator=>  OutDataTypeStr=boolean  RndMeth=Simplest
  Relational Operator1 : RelationalOperator  Operator=>  OutDataTypeStr=boolean  RndMeth=Simplest
  Relational Operator2 : RelationalOperator  Operator=>  OutDataTypeStr=boolean  RndMeth=Simplest
  Scope1 : Scope  NumInputPorts=2
  Scope2 : Scope  NumInputPorts=2
  Scope3 : Scope  NumInputPorts=2
  Scope4 : Scope  Commented=on  NumInputPorts=2
  Scope5 : Scope  Commented=on  NumInputPorts=2
  Scope6 : Scope
  Scope7 : Scope
  Scope8 : Scope
  Sum1 : Sum  Commented=on  Inputs=+|-
  Sum2 : Sum  Commented=on  Inputs=+|-
  Sum3 : Sum  Commented=on  Inputs=+|-
  Sum4 : Sum  Inputs=+|-
  Sum5 : Sum  Inputs=+|-
  To Workspace : ToWorkspace  Commented=on  VariableName=rLoc5  SaveFormat=Timeseries  SampleTime=tSampData
  To Workspace1 : ToWorkspace  Commented=on  VariableName=rLoc_bar5  SaveFormat=Timeseries  SampleTime=tSampData
  To Workspace10 : ToWorkspace  Commented=on  VariableName=atkFlag65  SaveFormat=Timeseries  SampleTime=tSampData
  To Workspace2 : ToWorkspace  Commented=on  VariableName=r45  SaveFormat=Timeseries  SampleTime=tSampData
  To Workspace3 : ToWorkspace  Commented=on  VariableName=r_bar45  SaveFormat=Timeseries  SampleTime=tSampData
  To Workspace4 : ToWorkspace  Commented=on  VariableName=r_bar65  SaveFormat=Timeseries  SampleTime=tSampData
  To Workspace7 : ToWorkspace  Commented=on  VariableName=r65  SaveFormat=Timeseries  SampleTime=tSampData
  To Workspace8 : ToWorkspace  Commented=on  VariableName=atkFlagLoc5  SaveFormat=Timeseries  SampleTime=tSampData
  To Workspace9 : ToWorkspace  Commented=on  VariableName=atkFlag45  SaveFormat=Timeseries  SampleTime=tSampData
  tag scope: atkFlag45=global, atkFlag65=global, atkFlagLoc5=global, r45=global, r65=global, rLoc5=global
  wires:
  [xhat5] -> Sum5/2
  Product5/1 -> [rLoc5]
  Sum5/1 -> Abs4/1
  [y5] -> Sum5/1
  Abs4/1 -> Product5/1
  [secondary] -> Product5/2
  Sum2/1 -> Abs1/1
  From2/1 -> Product1/2
  Gain1/1 -> Scope4/2, Sum2/2
  Product1/1 -> Goto7/1
  From7/1 -> Gain1/1
  Abs1/1 -> Product1/1
  From8/1 -> Scope4/1, Sum2/1
  Product2/1 -> Goto1/1
  From1/1 -> Product2/2
  From4/1 -> Scope5/1, Sum1/1
  From3/1 -> Gain2/1
  Sum1/1 -> Abs2/1
  Abs2/1 -> Product2/1
  Gain2/1 -> Sum1/2, Scope5/2
  Relational Operator1/1 -> Logical Operator1/1
  [rLoc_bar] -> Gain4/1
  Logical Operator1/1 -> To Workspace9/1, Scope7/1, [atkFlag45]
  [rLoc5] -> Relational Operator/1
  Relational Operator/1 -> Logical Operator/1
  [r_bar] -> Gain5/1
  Gain5/1 -> Relational Operator1/2
  Logical Operator/1 -> To Workspace8/1, Scope6/1, [atkFlagLoc5]
  [r45] -> Relational Operator1/1
  Relational Operator2/1 -> Logical Operator2/1
  Gain4/1 -> Relational Operator/2
  Gain6/1 -> Relational Operator2/2
  [r65] -> Relational Operator2/1
  [r_bar] -> Gain6/1
  Logical Operator2/1 -> To Workspace10/1, Scope8/1, [atkFlag65]
  Gain8/1 -> To Workspace4/1, Scope3/2
  [rLoc_bar] -> Gain3/1
  [r_bar] -> Gain8/1
  Gain3/1 -> To Workspace1/1, Scope2/2
  [r45] -> To Workspace2/1, Scope1/1
  [r_bar] -> Gain7/1
  Gain7/1 -> To Workspace3/1, Scope1/2
  [r65] -> To Workspace7/1, Scope3/1
  [rLoc5] -> To Workspace/1, Scope2/1
  From29/1 -> Product4/2
  From27/1 -> Sum3/2
  From28/1 -> Sum3/1
  Sum3/1 -> Abs3/1
  Product4/1 -> Gain9/1, Gain10/1
  Abs3/1 -> Product4/1
  Gain9/1 -> Goto2/1
  Gain10/1 -> Goto3/1
  Gain11/1 -> [r65]
  Gain12/1 -> [r45]
  Abs5/1 -> Product3/1
  Product3/1 -> Gain11/1, Gain12/1
  Sum4/1 -> Abs5/1
  [yComm5] -> Sum4/1
  [secondary] -> Product3/2
  Gain13/1 -> Sum4/2
  [xbar5] -> Gain13/1

== system simulation_w_switch_sln3/DGU5/Luenberger  Observer ==
  Gain1 : Gain  Gain=bigCyComm  Multiplication=Matrix(K*u) (u vector)
  Gain17 : Gain  Gain=[DGU(5).B , DGU(5).Li , DGU(5).M , Aij(4*n+1:5*n,:)]  Multiplication=Matrix(K*u) (u vector)
  Gain18 : Gain  Gain=DGU(5).A-DGU(5).Li*DGU(5).C  Multiplication=Matrix(K*u) (u vector)
  Integrator4 : Integrator  ExternalReset=rising  InitialConditionSource=external  InitialCondition=[0;0;0]
  Mux : Mux  Inputs=5
  Product4 : Product  Multiplication=Matrix(*)
  Sum10 : Sum  Inputs=++|
  tag scope: xhat5=global
  wires:
  Product4/1 -> [xhat5]
  [Il5] -> Mux/3
  [y5] -> Integrator4/3, Mux/2
  [Vref5] -> Mux/4
  Gain17/1 -> Sum10/2
  Gain18/1 -> Sum10/1
  [secondary] -> Integrator4/2, Product4/2
  Mux/1 -> Gain17/1
  Sum10/1 -> Integrator4/1
  Integrator4/1 -> Product4/1, Gain18/1
  [Vt5] -> Mux/1
  [yComm5] -> Gain1/1
  Gain1/1 -> Mux/5

== system simulation_w_switch_sln3/DGU5/Primary  Voltage  Controller ==
  Gain1 : Gain  Gain=DGU(5).K  Multiplication=Matrix(K*u) (u vector)
  tag scope: Vt5d=global
  wires:
  [y5] -> Gain1/1
  Gain1/1 -> [Vt5d]

== system simulation_w_switch_sln3/DGU5/Secondary Consensus Layer ==
  note: deltaV5
  Gain10 : Gain  Gain=length(DGU(5).Ni)
  Gain16 : Gain  Gain=DGU(5).kI
  Gain4 : Gain  Gain=repmat([0 0 0 0 1 0],1,6)  Multiplication=Matrix(K*u) (u vector)
  Integrator4 : Integrator  ExternalReset=rising
  Sum14 : Sum  Inputs=|+-
  Sum15 : Sum  Inputs=|++
  Switch4 : Switch  Criteria=u2 > Threshold  Threshold=0.1
  tag scope: Vref5=global
  wires:
  Gain16/1 -> Integrator4/1
  Sum14/1 -> Gain16/1
  Gain4/1 -> Sum14/1
  Sum15/1 -> Switch4/1
  [It5] -> Gain10/1
  Integrator4/1 -> Sum15/1
  Switch4/1 -> [Vref5]
  [Vref] -> Switch4/3, Sum15/2
  [yComm5] -> Gain4/1
  Gain10/1 -> Sum14/2
  [secondary] -> Switch4/2, Integrator4/2

== system simulation_w_switch_sln3/DGU5/Switching ==
  Divide : Product  Inputs=*/
  Logical Operator : Logic  Operator=NOT  AllPortsSameDT=off  OutDataTypeStr=boolean
  PWM Generator (DC-DC) : powerlib_meascontrol/Pulse & Signal Generators/PWM Generator (DC-DC)  Fsw=10000  Ts=0
  tag scope: SW_Buck_5=global, SW_Buck_5n=global, SW_Duty_5=global
  wires:
  [Vs5] -> Divide/2
  Logical Operator/1 -> [SW_Buck_5n]
  PWM Generator (DC-DC)/1 -> Logical Operator/1, [SW_Buck_5]
  Divide/1 -> [SW_Duty_5], PWM Generator (DC-DC)/1
  [Vt5d] -> Divide/1

== system simulation_w_switch_sln3/DGU5/UIO ==
  note: Single UIO for all neighbors of DGU 1 with Switched Inputs
  note: Calculated Switching Inputs
  note: 6x6 UIO for the states of DGUs with average dynamics
  Constant1 : Constant  Commented=on  Value=Vs
  Constant2 : Constant  Commented=on  Value=0.8132
  Divide : Product  Commented=on  Inputs=*/  Multiplication=Matrix(*)
  From5 : From  Commented=on  GotoTag=yComm5  TagVisibility=global
  From7 : From  Commented=on  GotoTag=yComm5  TagVisibility=global
  From8 : From  Commented=on  GotoTag=SW_yComm5  TagVisibility=global
  From9 : From  Commented=on  GotoTag=secondary  TagVisibility=global
  Gain15 : Gain  Gain=bH  Multiplication=Matrix(K*u) (u vector)
  Gain16 : Gain  Gain=inv(bC)-bH  Multiplication=Matrix(K*u) (u vector)
  Gain17 : Gain  Gain=bKhat  Multiplication=Matrix(K*u) (u vector)
  Gain18 : Gain  Gain=bF  Multiplication=Matrix(K*u) (u vector)
  Gain4 : Gain  Commented=on  Gain=K  Multiplication=Matrix(K*u) (u vector)
  Gain5 : Gain  Commented=on  Gain=[Khat T*B]  Multiplication=Matrix(K*u) (u vector)
  Gain6 : Gain  Commented=on  Gain=F  Multiplication=Matrix(K*u) (u vector)
  Gain7 : Gain  Commented=on  Gain=59.7999
  Gain8 : Gain  Commented=on  Gain=H  Multiplication=Matrix(K*u) (u vector)
  Gain9 : Gain  Commented=on  Gain=T  Multiplication=Matrix(K*u) (u vector)
  Goto : Goto  Commented=on  GotoTag=SW_yComm5  TagVisibility=global
  Goto3 : Goto  Commented=on  GotoTag=y_j5_hat  TagVisibility=global
  Goto4 : Goto  Commented=on  GotoTag=Duty_yComm5  TagVisibility=global
  Integrator1 : Integrator  Commented=on  ExternalReset=rising  InitialConditionSource=external
  Integrator4 : Integrator  ExternalReset=rising  InitialConditionSource=external  InitialCondition=[0;0;0]
  Mux3 : Mux  Commented=on  Inputs=2
  PWM Generator (DC-DC) : powerlib_meascontrol/Pulse & Signal Generators/PWM Generator (DC-DC)  Commented=on  Fsw=10000  Ts=0
  Product1 : Product  Commented=on  Multiplication=Matrix(*)
  Product4 : Product  Multiplication=Matrix(*)
  Sum10 : Sum  Inputs=++|
  Sum11 : Sum  Inputs=++|
  Sum2 : Sum  Commented=on  Inputs=++|
  Sum3 : Sum  Commented=on  Inputs=++|
  Sum4 : Sum  Commented=on  Inputs=|-+
  tag scope: xbar5=global
  wires:
  PWM Generator (DC-DC)/1 -> Goto/1
  Divide/1 -> Goto4/1, PWM Generator (DC-DC)/1
  Constant1/1 -> Divide/2
  Gain4/1 -> Divide/1
  From7/1 -> Gain4/1
  Constant2/1 -> Sum4/1
  From5/1 -> Gain8/1, Gain9/1, Mux3/1
  Sum3/1 -> Product1/1
  Gain5/1 -> Sum2/2
  Gain7/1 -> Sum4/2
  From8/1 -> Gain7/1
  Mux3/1 -> Gain5/1
  Gain8/1 -> Sum3/1
  Gain9/1 -> Integrator1/3
  From9/1 -> Integrator1/2, Product1/2
  Sum2/1 -> Integrator1/1
  Sum4/1 -> Mux3/2
  Integrator1/1 -> Sum3/2, Gain6/1
  Gain6/1 -> Sum2/1
  Product1/1 -> Goto3/1
  Sum11/1 -> Product4/1
  Gain17/1 -> Sum10/2
  Gain16/1 -> Integrator4/3
  Sum10/1 -> Integrator4/1
  [yComm5] -> Gain16/1, Gain15/1, Gain17/1
  Gain18/1 -> Sum10/1
  Gain15/1 -> Sum11/1
  Product4/1 -> [xbar5]
  Integrator4/1 -> Sum11/2, Gain18/1
  [secondary] -> Integrator4/2, Product4/2

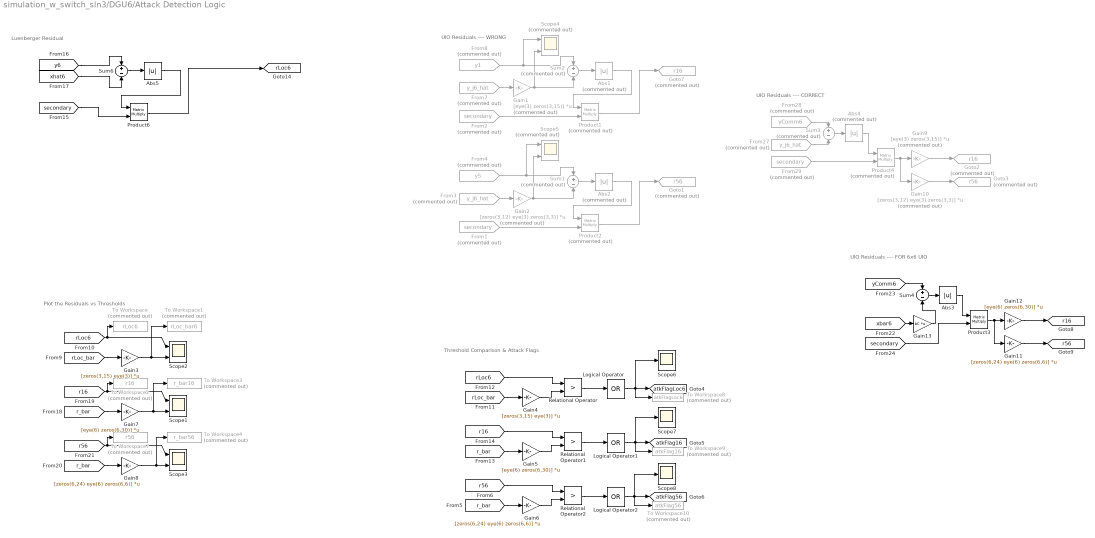
== system simulation_w_switch_sln3/DGU6/Attack Detection Logic ==
  note: UIO Residuals ---- WRONG
  note: Luenberger Residual
  note: Threshold Comparison & Attack Flags
  note: Plot the Residuals vs Thresholds
  note: UIO Residuals ---- CORRECT
  note: UIO Residuals ---- FOR 6x6 UIO
  Abs1 : Abs  Commented=on
  Abs2 : Abs  Commented=on
  Abs3 : Abs  ZeroCross=off
  Abs4 : Abs  Commented=on
  Abs5 : Abs
  From1 : From  Commented=on  GotoTag=secondary  TagVisibility=global
  From2 : From  Commented=on  GotoTag=secondary  TagVisibility=global
  From27 : From  Commented=on  GotoTag=y_j6_hat  TagVisibility=global
  From28 : From  Commented=on  GotoTag=yComm6  TagVisibility=global
  From29 : From  Commented=on  GotoTag=secondary  TagVisibility=global
  From3 : From  Commented=on  GotoTag=y_j6_hat  TagVisibility=global
  From4 : From  Commented=on  GotoTag=y5  TagVisibility=global
  From7 : From  Commented=on  GotoTag=y_j6_hat  TagVisibility=global
  From8 : From  Commented=on  GotoTag=y1  TagVisibility=global
  Gain1 : Gain  Commented=on  Gain=[eye(3) zeros(3,15)]  Multiplication=Matrix(K*u) (u vector)
  Gain10 : Gain  Commented=on  Gain=[zeros(3,12) eye(3) zeros(3,3)]  Multiplication=Matrix(K*u) (u vector)
  Gain11 : Gain  Gain=[zeros(6,24) eye(6) zeros(6,6)]  Multiplication=Matrix(K*u) (u vector)
  Gain12 : Gain  Gain=[eye(6) zeros(6,30)]  Multiplication=Matrix(K*u) (u vector)
  Gain13 : Gain  Gain=bC  Multiplication=Matrix(K*u) (u vector)
  Gain2 : Gain  Commented=on  Gain=[zeros(3,12) eye(3) zeros(3,3)]  Multiplication=Matrix(K*u) (u vector)
  Gain3 : Gain  Gain=[zeros(3,15) eye(3)]  Multiplication=Matrix(K*u) (u vector)
  Gain4 : Gain  Gain=[zeros(3,15) eye(3)]  Multiplication=Matrix(K*u) (u vector)
  Gain5 : Gain  Gain=[eye(6) zeros(6,30)]  Multiplication=Matrix(K*u) (u vector)
  Gain6 : Gain  Gain=[zeros(6,24) eye(6) zeros(6,6)]  Multiplication=Matrix(K*u) (u vector)
  Gain7 : Gain  Gain=[eye(6) zeros(6,30)]  Multiplication=Matrix(K*u) (u vector)
  Gain8 : Gain  Gain=[zeros(6,24) eye(6) zeros(6,6)]  Multiplication=Matrix(K*u) (u vector)
  Gain9 : Gain  Commented=on  Gain=[eye(3) zeros(3,15)]  Multiplication=Matrix(K*u) (u vector)
  Goto1 : Goto  Commented=on  GotoTag=r56  TagVisibility=global
  Goto2 : Goto  Commented=on  GotoTag=r16  TagVisibility=global
  Goto3 : Goto  Commented=on  GotoTag=r56  TagVisibility=global
  Goto7 : Goto  Commented=on  GotoTag=r16  TagVisibility=global
  Logical Operator : Logic  Operator=OR  Inputs=1  AllPortsSameDT=off  OutDataTypeStr=boolean
  Logical Operator1 : Logic  Operator=OR  Inputs=1  AllPortsSameDT=off  OutDataTypeStr=boolean
  Logical Operator2 : Logic  Operator=OR  Inputs=1  AllPortsSameDT=off  OutDataTypeStr=boolean
  Product1 : Product  Commented=on  Multiplication=Matrix(*)
  Product2 : Product  Commented=on  Multiplication=Matrix(*)
  Product3 : Product  Multiplication=Matrix(*)
  Product4 : Product  Commented=on  Multiplication=Matrix(*)
  Product6 : Product  Multiplication=Matrix(*)
  Relational Operator : RelationalOperator  Operator=>  OutDataTypeStr=boolean  RndMeth=Simplest
  Relational Operator1 : RelationalOperator  Operator=>  OutDataTypeStr=boolean  RndMeth=Simplest
  Relational Operator2 : RelationalOperator  Operator=>  OutDataTypeStr=boolean  RndMeth=Simplest
  Scope1 : Scope  NumInputPorts=2
  Scope2 : Scope  NumInputPorts=2
  Scope3 : Scope  NumInputPorts=2
  Scope4 : Scope  Commented=on  NumInputPorts=2
  Scope5 : Scope  Commented=on  NumInputPorts=2
  Scope6 : Scope
  Scope7 : Scope
  Scope8 : Scope
  Sum1 : Sum  Commented=on  Inputs=+|-
  Sum2 : Sum  Commented=on  Inputs=+|-
  Sum3 : Sum  Commented=on  Inputs=+|-
  Sum4 : Sum  Inputs=+|-
  Sum6 : Sum  Inputs=+|-
  To Workspace : ToWorkspace  Commented=on  VariableName=rLoc6  SaveFormat=Timeseries  SampleTime=tSampData
  To Workspace1 : ToWorkspace  Commented=on  VariableName=rLoc_bar6  SaveFormat=Timeseries  SampleTime=tSampData
  To Workspace10 : ToWorkspace  Commented=on  VariableName=atkFlag56  SaveFormat=Timeseries  SampleTime=tSampData
  To Workspace2 : ToWorkspace  Commented=on  VariableName=r16  SaveFormat=Timeseries  SampleTime=tSampData
  To Workspace3 : ToWorkspace  Commented=on  VariableName=r_bar16  SaveFormat=Timeseries  SampleTime=tSampData
  To Workspace4 : ToWorkspace  Commented=on  VariableName=r_bar56  SaveFormat=Timeseries  SampleTime=tSampData
  To Workspace7 : ToWorkspace  Commented=on  VariableName=r56  SaveFormat=Timeseries  SampleTime=tSampData
  To Workspace8 : ToWorkspace  Commented=on  VariableName=atkFlagLoc6  SaveFormat=Timeseries  SampleTime=tSampData
  To Workspace9 : ToWorkspace  Commented=on  VariableName=atkFlag16  SaveFormat=Timeseries  SampleTime=tSampData
  tag scope: atkFlag16=global, atkFlag56=global, atkFlagLoc6=global, r16=global, r56=global, rLoc6=global
  wires:
  Product6/1 -> [rLoc6]
  Sum6/1 -> Abs5/1
  [secondary] -> Product6/2
  [xhat6] -> Sum6/2
  [y6] -> Sum6/1
  Abs5/1 -> Product6/1
  Product1/1 -> Goto7/1
  From2/1 -> Product1/2
  From8/1 -> Scope4/1, Sum2/1
  From7/1 -> Gain1/1
  Sum2/1 -> Abs1/1
  Abs1/1 -> Product1/1
  Gain1/1 -> Scope4/2, Sum2/2
  Product2/1 -> Goto1/1
  From1/1 -> Product2/2
  From4/1 -> Scope5/1, Sum1/1
  From3/1 -> Gain2/1
  Sum1/1 -> Abs2/1
  Abs2/1 -> Product2/1
  Relational Operator1/1 -> Logical Operator1/1
  [rLoc_bar] -> Gain4/1
  Logical Operator1/1 -> Scope7/1, To Workspace9/1, [atkFlag16]
  [rLoc6] -> Relational Operator/1
  Relational Operator/1 -> Logical Operator/1
  [r_bar] -> Gain5/1
  Gain5/1 -> Relational Operator1/2
  Logical Operator/1 -> Scope6/1, To Workspace8/1, [atkFlagLoc6]
  [r16] -> Relational Operator1/1
  Relational Operator2/1 -> Logical Operator2/1
  Gain4/1 -> Relational Operator/2
  Gain6/1 -> Relational Operator2/2
  [r56] -> Relational Operator2/1
  [r_bar] -> Gain6/1
  Logical Operator2/1 -> To Workspace10/1, Scope8/1, [atkFlag56]
  [r_bar] -> Gain8/1
  Gain7/1 -> To Workspace3/1, Scope1/2
  [rLoc6] -> To Workspace/1, Scope2/1
  [r16] -> To Workspace2/1, Scope1/1
  [r56] -> To Workspace7/1, Scope3/1
  Gain3/1 -> To Workspace1/1, Scope2/2
  [r_bar] -> Gain7/1
  Gain8/1 -> To Workspace4/1, Scope3/2
  [rLoc_bar] -> Gain3/1
  Gain2/1 -> Scope5/2, Sum1/2
  From29/1 -> Product4/2
  From27/1 -> Sum3/2
  From28/1 -> Sum3/1
  Sum3/1 -> Abs4/1
  Product4/1 -> Gain9/1, Gain10/1
  Abs4/1 -> Product4/1
  Gain9/1 -> Goto2/1
  Gain10/1 -> Goto3/1
  Gain11/1 -> [r56]
  Gain12/1 -> [r16]
  Abs3/1 -> Product3/1
  Product3/1 -> Gain11/1, Gain12/1
  Sum4/1 -> Abs3/1
  [yComm6] -> Sum4/1
  [secondary] -> Product3/2
  [xbar6] -> Gain13/1
  Gain13/1 -> Sum4/2

== system simulation_w_switch_sln3/DGU6/Luenberger  Observer1 ==
  Gain1 : Gain  Gain=bigCyComm  Multiplication=Matrix(K*u) (u vector)
  Gain17 : Gain  Gain=[DGU(6).B , DGU(6).Li , DGU(6).M , Aij(5*n+1:6*n,:)]  Multiplication=Matrix(K*u) (u vector)
  Gain18 : Gain  Gain=DGU(6).A-DGU(6).Li*DGU(6).C  Multiplication=Matrix(K*u) (u vector)
  Integrator4 : Integrator  ExternalReset=rising  InitialConditionSource=external  InitialCondition=[0;0;0]
  Mux : Mux  Inputs=5
  Product4 : Product  Multiplication=Matrix(*)
  Sum10 : Sum  Inputs=++|
  tag scope: xhat6=global
  wires:
  Product4/1 -> [xhat6]
  [Il6] -> Mux/3
  [y6] -> Integrator4/3, Mux/2
  [Vref6] -> Mux/4
  Gain17/1 -> Sum10/2
  Gain18/1 -> Sum10/1
  [secondary] -> Integrator4/2, Product4/2
  Mux/1 -> Gain17/1
  Sum10/1 -> Integrator4/1
  Integrator4/1 -> Product4/1, Gain18/1
  [Vt6] -> Mux/1
  [yComm6] -> Gain1/1
  Gain1/1 -> Mux/5

== system simulation_w_switch_sln3/DGU6/Primary  Voltage  Controller ==
  Gain1 : Gain  Gain=DGU(6).K  Multiplication=Matrix(K*u) (u vector)
  tag scope: Vt6d=global
  wires:
  [y6] -> Gain1/1
  Gain1/1 -> [Vt6d]

== system simulation_w_switch_sln3/DGU6/Secondary Consensus Layer ==
  note: deltaV6
  Gain11 : Gain  Gain=length(DGU(6).Ni)
  Gain17 : Gain  Gain=DGU(6).kI
  Gain5 : Gain  Gain=repmat([0 0 0 0 1 0],1,6)  Multiplication=Matrix(K*u) (u vector)
  Integrator5 : Integrator  ExternalReset=rising
  Sum16 : Sum  Inputs=|+-
  Sum17 : Sum  Inputs=|++
  Switch5 : Switch  Criteria=u2 > Threshold  Threshold=0.1
  tag scope: Vref6=global
  wires:
  Switch5/1 -> [Vref6]
  Integrator5/1 -> Sum17/1
  Sum16/1 -> Gain17/1
  Gain11/1 -> Sum16/2
  [Vref] -> Switch5/3, Sum17/2
  Gain17/1 -> Integrator5/1
  Gain5/1 -> Sum16/1
  [secondary] -> Integrator5/2, Switch5/2
  [It6] -> Gain11/1
  Sum17/1 -> Switch5/1
  [yComm6] -> Gain5/1

== system simulation_w_switch_sln3/DGU6/Switching ==
  Divide : Product  Inputs=*/
  Logical Operator : Logic  Operator=NOT  AllPortsSameDT=off  OutDataTypeStr=boolean
  PWM Generator (DC-DC) : powerlib_meascontrol/Pulse & Signal Generators/PWM Generator (DC-DC)  Fsw=10000  Ts=0
  tag scope: SW_Buck_6=global, SW_Buck_6n=global, SW_Duty_6=global
  wires:
  [Vs6] -> Divide/2
  Logical Operator/1 -> [SW_Buck_6n]
  PWM Generator (DC-DC)/1 -> Logical Operator/1, [SW_Buck_6]
  Divide/1 -> [SW_Duty_6], PWM Generator (DC-DC)/1
  [Vt6d] -> Divide/1
